simulink model "simulink1"  (R2021a)
settings: Solver=VariableStepAuto  StartTime=0.0  StopTime=10.0  RelTol=1e-3
settings Model: Creator=student  LastModifiedBy=НОРД
settings SolverCC: AlgebraicLoopSolver=TrustRegion
settings DataIOCC: ReturnWorkspaceOutputs=off
settings DebuggingCC: SFMachineParentedDataDiag=warning  ArithmeticOperatorsInVariantConditions=warning
settings SFSimCC: CustomCodeUndefinedFunction=UseInterfaceOnly

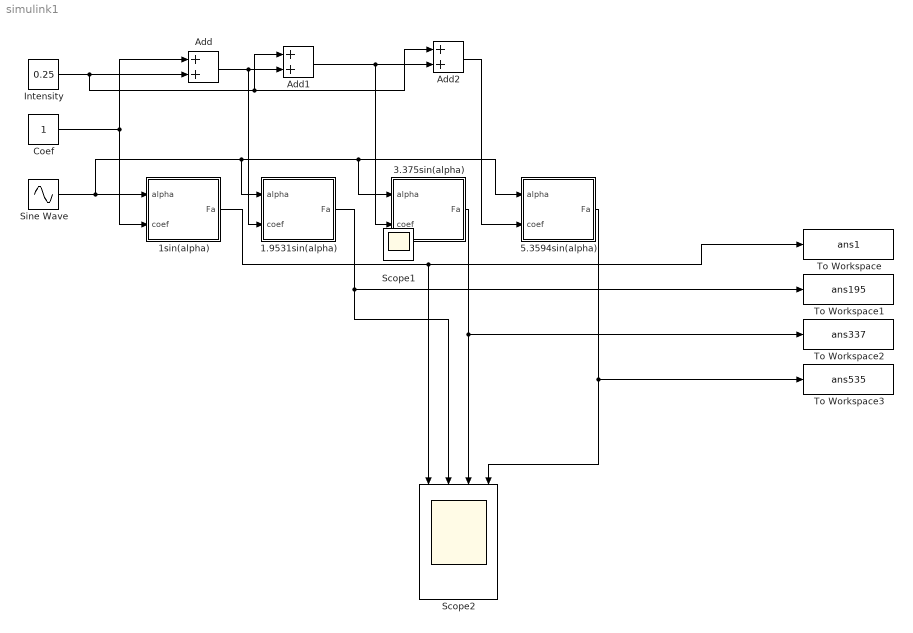
== system simulink1 ==
  1.9531sin(alpha) : Subsystem
  1sin(alpha) : Subsystem
  3.375sin(alpha) : Subsystem
  5.3594sin(alpha) : Subsystem
  Add : Sum
  Add1 : Sum
  Add2 : Sum
  "Coef " : Constant
  "Intensity " : Constant  Value=0.25
  Scope2 : Scope  NumInputPorts=4
  Sine Wave : Sin  SampleTime=0
  To Workspace : ToWorkspace  VariableName=ans1  SampleTime=-1
  To Workspace1 : ToWorkspace  VariableName=ans195  SampleTime=-1
  To Workspace2 : ToWorkspace  VariableName=ans337  SampleTime=-1
  To Workspace3 : ToWorkspace  VariableName=ans535  SampleTime=-1
  Scope1 : Scope
  wires:
  "Coef "/1 -> 1sin(alpha)/2(coef), Add/1
  Add/1 -> Add1/2, 1.9531sin(alpha)/2(coef)
  Add2/1 -> 5.3594sin(alpha)/2(coef)
  1.9531sin(alpha)/1(Fa) -> Scope2/2, To Workspace1/1
  "Intensity "/1 -> Add2/1, Add1/1, Add/2
  Add1/1 -> 3.375sin(alpha)/2(coef), Add2/2
  3.375sin(alpha)/1(Fa) -> Scope2/3, To Workspace2/1
  5.3594sin(alpha)/1(Fa) -> Scope2/4, To Workspace3/1
  Sine Wave/1 -> 1sin(alpha)/1(alpha), 3.375sin(alpha)/1(alpha), 5.3594sin(alpha)/1(alpha), 1.9531sin(alpha)/1(alpha)
  1sin(alpha)/1(Fa) -> To Workspace/1, Scope2/1

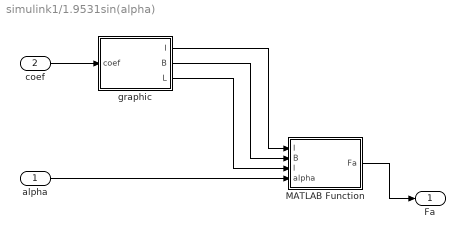
== system simulink1/1.9531sin(alpha) ==
  alpha : Inport
  coef : Inport  Port=2
  MATLAB Function : MATLAB Function  TreatAsAtomicUnit=on
  graphic : MATLAB Function  TreatAsAtomicUnit=on
  Fa : Outport
  wires:
  coef/1 -> graphic/1(coef)
  graphic/1(I) -> MATLAB Function/1(I)
  alpha/1 -> MATLAB Function/4(alpha)
  graphic/2(B) -> MATLAB Function/2(B)
  graphic/3(L) -> MATLAB Function/3(l)
  MATLAB Function/1(Fa) -> Fa/1

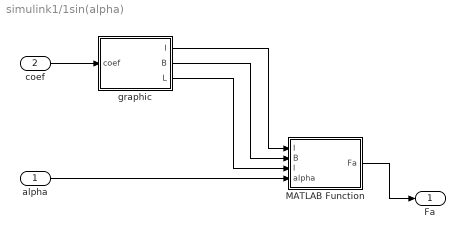
== system simulink1/1sin(alpha) ==
  alpha : Inport
  coef : Inport  Port=2
  MATLAB Function : MATLAB Function  TreatAsAtomicUnit=on
  graphic : MATLAB Function  TreatAsAtomicUnit=on
  Fa : Outport
  wires:
  coef/1 -> graphic/1(coef)
  graphic/1(I) -> MATLAB Function/1(I)
  alpha/1 -> MATLAB Function/4(alpha)
  graphic/2(B) -> MATLAB Function/2(B)
  graphic/3(L) -> MATLAB Function/3(l)
  MATLAB Function/1(Fa) -> Fa/1

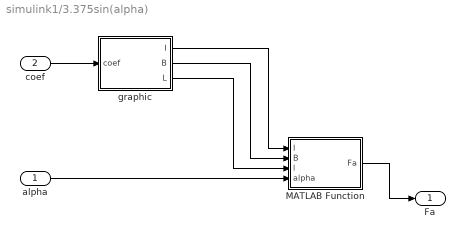
== system simulink1/3.375sin(alpha) ==
  alpha : Inport
  coef : Inport  Port=2
  MATLAB Function : MATLAB Function  TreatAsAtomicUnit=on
  graphic : MATLAB Function  TreatAsAtomicUnit=on
  Fa : Outport
  wires:
  coef/1 -> graphic/1(coef)
  graphic/1(I) -> MATLAB Function/1(I)
  alpha/1 -> MATLAB Function/4(alpha)
  graphic/2(B) -> MATLAB Function/2(B)
  graphic/3(L) -> MATLAB Function/3(l)
  MATLAB Function/1(Fa) -> Fa/1

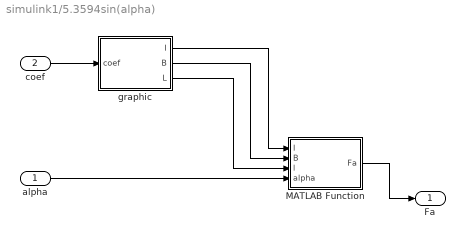
== system simulink1/5.3594sin(alpha) ==
  alpha : Inport
  coef : Inport  Port=2
  MATLAB Function : MATLAB Function  TreatAsAtomicUnit=on
  graphic : MATLAB Function  TreatAsAtomicUnit=on
  Fa : Outport
  wires:
  coef/1 -> graphic/1(coef)
  graphic/1(I) -> MATLAB Function/1(I)
  alpha/1 -> MATLAB Function/4(alpha)
  graphic/2(B) -> MATLAB Function/2(B)
  graphic/3(L) -> MATLAB Function/3(l)
  MATLAB Function/1(Fa) -> Fa/1

== matlab function simulink1/3.375sin(alpha)/MATLAB Function ==
  data: I input; Fa output; B input; l input; alpha input
function Fa = amperforce(I,B,l,alpha)
Fa = I.*B.*l.*alpha;
end

== matlab function simulink1/5.3594sin(alpha)/MATLAB Function ==
  data: I input; Fa output; B input; l input; alpha input
function Fa = amperforce(I,B,l,alpha)
Fa = I.*B.*l.*alpha;
end

== matlab function simulink1/1sin(alpha)/MATLAB Function ==
  data: I input; Fa output; B input; l input; alpha input
function Fa = amperforce(I,B,l,alpha)
Fa = I.*B.*l.*alpha;
end

== matlab function simulink1/1sin(alpha)/graphic ==
  data: I output; coef input; B output; L output
function [I,B,L] = graphic(coef)
I = 1*coef;
B = 2*coef;
L = 0.5*coef;
end

== matlab function simulink1/1.9531sin(alpha)/MATLAB Function ==
  data: I input; Fa output; B input; l input; alpha input
function Fa = amperforce(I,B,l,alpha)
Fa = I.*B.*l.*alpha;
end

== matlab function simulink1/1.9531sin(alpha)/graphic ==
  data: I output; coef input; B output; L output
function [I,B,L] = graphic(coef)
I = 1*coef;
B = 2*coef;
L = 0.5*coef;
end

== matlab function simulink1/3.375sin(alpha)/graphic ==
  data: I output; coef input; B output; L output
function [I,B,L] = graphic(coef)
I = 1*coef;
B = 2*coef;
L = 0.5*coef;
end

== matlab function simulink1/5.3594sin(alpha)/graphic ==
  data: I output; coef input; B output; L output
function [I,B,L] = graphic(coef)
I = 1*coef;
B = 2*coef;
L = 0.5*coef;
end
